simulink model "AUAV3_WITH_SLUGS_SENSOR_AND_CONTROLLER"  (Simulink 8.5)
settings: Solver=FixedStepDiscrete  StartTime=0.0  StopTime=10.0  FixedStep=T  RelTol=1e-3
PreLoadFcn:
  | T = 0.0025;
  | MavlinkBus;
  | 
  | % Baro Altitude Computation
  | % =========================
  | basePressure = 98192.64;
  | baseTemp = 288.215;
  | lapseRate = -0.00198122;
  | baseHeight = 0;
  | 
  | mcuInit
values from neighbouring files (symbols this model uses):
  apSampleTime = 0.01    [mcuInit.m]
  latlong_WP = 1    [mcuInit.m]
  mavlink_gps_raw_int_t = Simulink.Bus    [MavlinkBus.m]    (also in MavlinkBusMarcello.m)
  mavlink_raw_imu_t = Simulink.Bus    [MavlinkBus.m]    (also in MavlinkBusMarcello.m)
  mavlink_scaled_pressure_t = Simulink.Bus    [MavlinkBus.m]    (also in MavlinkBusMarcello.m)
  mavlink_sys_status_t = Simulink.Bus    [MavlinkBus.m]    (also in MavlinkBusMarcello.m)
  Xpoints = [0 0]    [mcuInit.m]
  Ypoints = [0 0]    [mcuInit.m]
  Zpoints = [0 0]    [mcuInit.m]
undefined symbols (not defined in the file or in its folder): A0, A14, A15, A2, A3, A5, A6, accBiasRateLimit, altLatLon, B0, bankCommandLimit, barAdjust, baroCutoff, baroCutTemp, C3, cubeAccelGain16405, cubeGyroGain16405, cubeMagGain16405, D0, D11, D13, D8, daLimit, data, daTrimMax, daTrimMin, deLimit, deTrimMax, deTrimMin, drLimit, drTrimMax, drTrimMin, dtLimit, dtTrimMax, dtTrimMin, F2, F3, G0, G15, gaind, GS_location, gyroBiasRateLimit, IC1max, IPStar, ISA_g, maxAcc, MaxDwnPthStar, maxDynPressure, maxEta, OC1max, P112, P127, P16, P21, P30, P31, P51, P64, P72, P75 ... (+39)
undefined symbols (not defined in the file): baroOffset, baroScale, barTGain1, barTGain2, barTMean1, barTMean2, bda, bde, bdr, bdt, bICda, bICde, bICdr, bICdt, derivativesConstant, lowRateSensorCutoff, mainSensorCutoff, mda, mde, mdr, mdt, mICda, mICde, mICdr, mICdt, pitotOffset, pitotScale, pitTGain1, pitTGain2, pitTMean1, pitTMean2, powerOffset, powerScale, pressureSensorCutoff, tempOffset, tempScale, vzCutoff, xCutoff, yCutoff
libraries: MCHP_Blockset x147, simulink x78, SLUGS_Library x31, aerolibconvert2 x6, aerolibutil x4, aerolibtransform2 x3, dspmtrx3 x2, aerolibobsolete x2
(part 3 of 12)

== system AUAV3_WITH_SLUGS_SENSOR_AND_CONTROLLER/Servo In Out ==
  Bias : Bias  Bias=-round(IC1max/2)
  Bias1 : Bias  Bias=-round(IC1max/2)
  Bias2 : Bias  Bias=+round(IC1max/2)
  Bias3 : Bias  Bias=+round(IC1max/2)
  Data Type Conversion2 : DataTypeConversion  OutDataTypeStr=uint16  ConvertRealWorld=Stored Integer (SI)  RndMeth=Simplest
  Data Type Conversion3 : DataTypeConversion  OutDataTypeStr=uint16  ConvertRealWorld=Stored Integer (SI)  RndMeth=Simplest
  Data Type Conversion4 : DataTypeConversion  OutDataTypeStr=int16  ConvertRealWorld=Stored Integer (SI)  RndMeth=Simplest
  Data Type Conversion5 : DataTypeConversion  OutDataTypeStr=int16  ConvertRealWorld=Stored Integer (SI)  RndMeth=Simplest
  Input Capture RC Receiver1 : MCHP_Blockset/Pulse Input//Output/Input Capture  IntPriority=7  Channel="[1     2     3     4     5     6]"  Channel_OLD="[1  2  3  4  5  6]"  PIN_IC1=Dynamic Options  PIN_IC1_TXT=D0 / P64 / Pin[72]  PIN_IC2=Dynamic Options  PIN_IC2_TXT=D8 / P72 / Pin[68]  PIN_IC3=Dynamic Options  PIN_IC3_TXT=D11 / P75 / Pin[71]  PIN_IC4=Dynamic Options  PIN_IC4_TXT=A15 / P31 / Pin[67]  PIN_IC5=Dynamic Options  PIN_IC5_TXT=A5 / P21 / Pin[61]  PIN_IC6=Dynamic Options  PIN_IC6_TXT=A14 / P30 / Pin[66]  PIN_IC7=Dynamic Options  PIN_IC7_TXT=A0 / P16 / Pin[17]  PIN_IC8=Dynamic Options  PIN_IC8_TXT=A0 / P16 / Pin[17]  PIN_IC9=Dynamic Options  PIN_IC9_TXT=A0 / P16 / Pin[17]  PIN_IC10=Dynamic Options  PIN_IC10_TXT=A0 / P16 / Pin[17]  PIN_IC11=Dynamic Options  PIN_IC11_TXT=A0 / P16 / Pin[17]  PIN_IC12=Dynamic Options  PIN_IC12_TXT=A0 / P16 / Pin[17]  PIN_IC13=Dynamic Options  PIN_IC13_TXT=A0 / P16 / Pin[17]  PIN_IC14=Dynamic Options  PIN_IC14_TXT=A0 / P16 / Pin[17]  PIN_IC15=Dynamic Options  PIN_IC15_TXT=A0 / P16 / Pin[17]  PIN_IC16=Dynamic Options  PIN_IC16_TXT=A0 / P16 / Pin[17]  Channel_UP_Down_Periode="[1     1     1     1     1     1]"  MaxChannel="[0.003   0.003   0.003   0.003   0.003   0.003]"  SafeMarge="[0     0     0     0     0     0]"  MaxChannelValue="2.^[ 14.680  14.680  14.680  14.680  14.680  14.680]  =>  [26249  26249  26249  26249  26249  26249]"  ICxmax="[26249  26249  26249  26249  26249  26249]"  Timer="[1  1  1  1  1  1]"  ChangeDetected="[0     0     0     0     0     0]"  ChangeDetectedPortRef=3  SampleTime=.01  Status=OK  MCHP_PORT={Input Capture 1}{IC1}6:0:P64;{Input Capture 2}{IC2}6:0:P72;{Input Capture 3}{IC3}6:0:P75;{Input Capture 4}{IC4}6:0:P31;{Input Capture 5}{IC5}6:0:P21;{Input Capture 6}{IC6}6:0:P30;  MCHP_TIMER_REQUEST="{Input Capture 1}{IC1}6:0:1:0:[1  2  3  4  5]:210000;{Input Capture 1}{IC1}6:0:1:0:[1  2  3  4  5]:210000;{Input Capture 1}{IC1}6:0:1:0:[1  2  3  4  5]:210000;{Input Capture 1}{IC1}6:0:1:0:[1  2  3  4  5]:210000;{Input Capture 1}{IC1}6:0:1:0:[1  2  3  4  5]:210000;{Input Capture 1}{IC1}6:0:1:0:[1  2  3  4  5]:210000;"  MCHP_TIMER_RESULT=[1 26249.000000000011 ;1 26249.000000000011 ;1 26249.000000000011 ;1 26249.000000000011 ;1 26249.000000000011 ;1 26249.000000000011 ]  MCHP_MASTERLINK=|
      | AUAV3_WITH_SLUGS_SENSOR_AND_CONTROLLER/Microchip Master
      | AUAV V3 Board
      | Busy Flag on D2 (RA6)
  Mixing : Subsystem
  Output Compare - HW Drive Servo motor : MCHP_Blockset/Pulse Input//Output/Output Compare - HW  Channel="[1     2]"  Channel_OLD="[1     2]"  PIN_OC1=Dynamic Options  PIN_OC1_TXT=G0 / P112 / Pin[90]  PIN_OC2=Dynamic Options  PIN_OC2_TXT=E0 / P80 / Pin[93]  PIN_OC3=Dynamic Options  PIN_OC3_TXT=D0 / P64 / Pin[72]  PIN_OC4=Dynamic Options  PIN_OC4_TXT=D0 / P64 / Pin[72]  PIN_OC5=Dynamic Options  PIN_OC5_TXT=D0 / P64 / Pin[72]  PIN_OC6=Dynamic Options  PIN_OC6_TXT=D0 / P64 / Pin[72]  PIN_OC7=Dynamic Options  PIN_OC7_TXT=D0 / P64 / Pin[72]  PIN_OC8=Dynamic Options  PIN_OC8_TXT=D0 / P64 / Pin[72]  PIN_OC9=Dynamic Options  PIN_OC9_TXT=D0 / P64 / Pin[72]  PIN_OC10=Dynamic Options  PIN_OC10_TXT=D0 / P64 / Pin[72]  PIN_OC11=Dynamic Options  PIN_OC11_TXT=D0 / P64 / Pin[72]  PIN_OC12=Dynamic Options  PIN_OC12_TXT=D0 / P64 / Pin[72]  PIN_OC13=Dynamic Options  PIN_OC13_TXT=D0 / P64 / Pin[72]  PIN_OC14=Dynamic Options  PIN_OC14_TXT=D0 / P64 / Pin[72]  PIN_OC15=Dynamic Options  PIN_OC15_TXT=D0 / P64 / Pin[72]  PIN_OC16=Dynamic Options  PIN_OC16_TXT=D0 / P64 / Pin[72]  PIN_OCFA=Dynamic Options  PIN_OCFA_TXT=A0 / P16 / Pin[17]  PIN_OCFB=Dynamic Options  PIN_OCFB_TXT=A0 / P16 / Pin[17]  PIN_OCFC=Dynamic Options  PIN_OCFC_TXT=A0 / P16 / Pin[17]  Channel_UP_Down_Periode="[5     5]"  PulseTrig=Single pulse triggered by block execution  InputPeriod=are set to the Max time (constant below)  MaxChannel="[0.003   0.003]"  MaxChannelUnique=.0001  MaxChannelValue="2.^[ 14.680  14.680]  =>  [26249  26249]"  OCxmax="[26249  26249]"  Timer="[1  1]"  SampleTime=.01  MCHP_PORT={Output Compare 1}{OC1}7:1:P112;{Output Compare 2}{OC2}7:1:P80;  MCHP_TIMER_REQUEST="{Output Compare 1}{OC1}7:0:1:0:[1  2  3  4  5]:210000;{Output Compare 1}{OC1}7:0:1:0:[1  2  3  4  5]:210000;"  MCHP_TIMER_RESULT=[1 26249.000000000011 ;1 26249.000000000011 ]  MCHP_MASTERLINK=|
      | AUAV3_WITH_SLUGS_SENSOR_AND_CONTROLLER/Microchip Master
      | AUAV V3 Board
      | Busy Flag on D2 (RA6)
  Saturation : Saturate  UpperLimit=OC1max*2.2/3  LowerLimit=OC1max*0.8/3  RndMeth=Simplest
  Saturation1 : Saturate  UpperLimit=OC1max*2.2/3  LowerLimit=OC1max*0.8/3  RndMeth=Simplest
  Out1 : Outport
  Out2 : Outport  Port=2
  Out3 : Outport  Port=3
  Out4 : Outport  Port=4
  wires:
  Input Capture RC Receiver1/1 -> Data Type Conversion4/1  "cmd PITCH raw"
  Input Capture RC Receiver1/4 -> Data Type Conversion5/1  "cmd ROLL raw"
  Bias/1 -> Mixing/1(Pitch)
  Bias1/1 -> Mixing/2(Roll)
  Bias2/1 -> Data Type Conversion2/1
  Bias3/1 -> Data Type Conversion3/1
  Saturation1/1 -> Output Compare - HW Drive Servo motor/2
  Saturation/1 -> Output Compare - HW Drive Servo motor/1
  Mixing/2(Cmd Servo Right) -> Bias3/1
  Mixing/1(Cmd Servo Left) -> Bias2/1
  Data Type Conversion4/1 -> Bias/1
  Data Type Conversion5/1 -> Bias1/1
  Data Type Conversion3/1 -> Saturation1/1
  Data Type Conversion2/1 -> Saturation/1
  Input Capture RC Receiver1/2 -> Out1/1
  Input Capture RC Receiver1/3 -> Out2/1
  Input Capture RC Receiver1/5 -> Out3/1
  Input Capture RC Receiver1/6 -> Out4/1

== system AUAV3_WITH_SLUGS_SENSOR_AND_CONTROLLER/Trim Vals [updated 4.28.16] ==
  Bufffer IC : Subsystem
  Control Surfaces [dT dA dR dE] : Selector  InputPortWidth=5  Indices=[1 2 4 3]
  Control Surface Input : Subsystem
  "Convert to Microseconds " : Subsystem
  Detect Transition High to Low : Subsystem
  Failsafe : Selector  InputPortWidth=5  Indices=[5]
  Grab I.C. : Subsystem  TreatAsAtomicUnit=on
  Manual or Auto? [navSupport.c] [updated 4.28.16] : MCHP_Blockset/User Functions/C Function Call  ParseFilesChkbx=off  ListFunctions1=Custom Function  Function1=extern uint8_T isApManual(uint16_T u1);  AddHeaderDeclaration=on  Function1Type=when block is updated (default)  FctReturnBlockOut=on  Fct1BlockOut=y1  DataCollected=0  ORDERING=None  SampleTime=-1  MCHP_MASTERLINK=|  PinDigitalInput=[]  PinDigitalOutput=[]  PinAnalogInput=[]
      | AUAV3_WITH_SLUGS_SENSOR_AND_CONTROLLER/Microchip Master
      | AUAV V3 Board
      | Busy Flag on D2 (RA6)
  Mean Filter the Transition : Subsystem
  dT Trim : Outport
  dA Trim : Outport  Port=2
  dR Trim : Outport  Port=3
  dE Trim : Outport  Port=4
  Pil Console : Outport  Port=5
  Manual? : Outport  Port=6
  V/I Sensor : Outport  Port=7
  wires:
  Manual or Auto? [navSupport.c] [updated 4.28.16]/1 -> Detect Transition High to Low/1(Switch), Manual?/1
  Control Surface Input/1(Pilot Console) -> Control Surfaces [dT dA dR dE]/1, Failsafe/1
  Control Surfaces [dT dA dR dE]/1 -> Pil Console/1, Bufffer IC/1(Pilot Console)
  Bufffer IC/1(dT_buf) -> Grab I.C./1(dT_buf)
  Bufffer IC/2(dA_buf) -> Grab I.C./2(dA_buf)
  Bufffer IC/3(dR_buf) -> Grab I.C./3(dR_buf)
  Bufffer IC/4(dE_buf) -> Grab I.C./4(dE_buf)
  Grab I.C./4(dE_trim (rad)) -> dE Trim/1
  Grab I.C./3(dR_trim (rad)) -> dR Trim/1
  Grab I.C./2(dA_trim (rad)) -> dA Trim/1
  Grab I.C./1(dT_trim (abs)) -> dT Trim/1
  Detect Transition High to Low/1(Transition) -> Grab I.C./Enable
  Failsafe/1 -> "Convert to Microseconds "/1(IC)
  "Convert to Microseconds "/1(uS) -> Mean Filter the Transition/1(Failsafe)
  Control Surface Input/2(Voltage/Current Sensor) -> V/I Sensor/1
  Mean Filter the Transition/1(filtered) -> Manual or Auto? [navSupport.c] [updated 4.28.16]/1

== system AUAV3_WITH_SLUGS_SENSOR_AND_CONTROLLER/Update PWM Commands and Send Telemetry [updated 4.27.16] ==
  PWM(rad) [dT dA dR dE] : Inport
  Pilot Console (IC) [dT dA dR dE] : Inport  Port=2
  Euler_rot : Inport  Port=3
  PQR_rot : Inport  Port=4
  Manual? : Inport  Port=5
  VI : Inport  Port=6
  Convert to Microseconds : Subsystem
  Create Telemetry Sentence [mavlinkCommsControlMcu.c] : MCHP_Blockset/User Functions/C Function Call  ParseFilesChkbx=off  ListFunctions1=Custom Function  Function1=extern void prepareTelemetryMavlink(uint8_T* y1);  AddHeaderDeclaration=on  Function1Type=when block is updated (default)  FctReturnBlockOut=on  Fct1BlockOut=y1  DataCollected=0  ORDERING=Input  SampleTime=0.04  MCHP_MASTERLINK=|  PinDigitalInput=[]  PinDigitalOutput=[]  PinAnalogInput=[]
      | AUAV3_WITH_SLUGS_SENSOR_AND_CONTROLLER/Microchip Master
      | AUAV V3 Board
      | Busy Flag on D2 (RA6)
  Demux : Demux
  Generate PWM Signals Based on the Control Type : Subsystem
  Navigation Mode [navSupport.c] : MCHP_Blockset/User Functions/C Function Call  ParseFilesChkbx=off  ListFunctions1=Custom Function  Function1=extern uint8_T getNavMode();  AddHeaderDeclaration=on  Function1Type=when block is updated (default)  FctReturnBlockOut=on  DataCollected=0  ORDERING=None  SampleTime=0.01  MCHP_MASTERLINK=|  PinDigitalInput=[]  PinDigitalOutput=[]  PinAnalogInput=[]
      | AUAV3_WITH_SLUGS_SENSOR_AND_CONTROLLER/Microchip Master
      | AUAV V3 Board
      | Busy Flag on D2 (RA6)
  PWM High Speed : MCHP_Blockset/PWM IO/PWM High Speed  pop1=[1]  chk1="[1  1  1  0]"  chkHL1="[1  1  1  1  0  0  1 ; 1  1  1  1  0  0  1]"  maxP1="[0.001       0.001       0.001       0.001       0.001       0.001       0.001 ; 0.001       0.001      1e-006       0.001       0.001       0.001       0.001]"  InitP2="[0.001       0.001       0.001       0.001       0.001       0.001       0.001 ; 0.001       0.001       0.001       0.001       0.001       0.001       0.001]"  chkP2="[0  0  0  0  1  1  1 ; 1  0  0  1  1  1  1]"  InitDC="[0.0005       0.0004       0.0003        0.001        0.001        0.001           50 ; 0.001        0.001        0.001        0.001        0.001        0.001           50]"  chkDC="[1  1  1  1  1  1  1 ; 0  0  0  1  1  1  1]"  InitPh="[0           0           0       0.001       0.001       0.001       0.001 ; 0           0           0       0.001       0.001       0.001       0.001]"  chkPh="[0  0  0  1  1  1  1 ; 0  0  0  1  1  1  1]"  edSEvTrigx={'0.0006','-1','-1','-1','-1','-1','-1'}  chkSEvTrigx="[0  0  0  0  1  1  1]"  popFlt="[1  1  1  1  1  1  1]"  popFltPin="[48  48  48  48  48  48  48]"  popFltPinRp="[1  1  1  1  1  1  1]"  popFltActivH="[1  2  1  1  1  1  1]"  popFltForceH="[2  2  2  2  2  2  2]"  popFltForceL="[1  1  1  1  1  1  1]"  chkFltBlkOut="[0  0  0  0  0  0  0]"  popDT="[3  3  3  3  3  3  3]"  edDTRx="[0.02      1e-005       0.001      1e-005      1e-005      1e-005      1e-005]"  edAltDTRx="[1e-005      0.0001      1e-005      1e-005      1e-005      1e-005      1e-005]"  S_INPUT="[5  5  5  5]"  S_OUTPUT=[]  ADC_VARTRIG={PWM Generator 1 Primary Trigger;1}{PWM Generator 2 Primary Trigger;3}{PWM Generator 3 Primary Trigger;5}{PWM Generator 4 Primary Trigger;7}  SampleTime=-1  ORDERING=None  MCHP_PORT={PWM1H}{PWM1H}4:4:E0;{PWM1L}{PWM1L}4:4:E1;{PWM2H}{PWM2H}4:4:E2;{PWM2L}{PWM2L}4:4:E3;{PWM3H}{PWM3H}4:4:E4;{PWM3L}{PWM3L}4:4:E5;{PWM4H}{PWM4H}4:4:E6;{PWM4L}{PWM4L}4:4:E7;  MCHP_MASTERLINK=|
      | AUAV3_WITH_SLUGS_SENSOR_AND_CONTROLLER/Microchip Master
      | AUAV V3 Board
      | Busy Flag on D2 (RA6)
  Rate Transition : RateTransition
  Send Data to Radio Modem [mavlinkCommsControlMcu.c] : MCHP_Blockset/User Functions/C Function Call  ParseFilesChkbx=off  ListFunctions1=Custom Function  Function1=extern void send2GS(uint8_T* u1);  AddHeaderDeclaration=on  Function1Type=when block is updated (default)  FctReturnBlockOut=on  Fct1BlockOut=y1  DataCollected=0  ORDERING=None  SampleTime=0.04  MCHP_MASTERLINK=|  PinDigitalInput=[]  PinDigitalOutput=[]  PinAnalogInput=[]
      | AUAV3_WITH_SLUGS_SENSOR_AND_CONTROLLER/Microchip Master
      | AUAV V3 Board
      | Busy Flag on D2 (RA6)
  Update Euler Angles [updateControlMcu.c] : MCHP_Blockset/User Functions/C Function Call  ParseFilesChkbx=off  ListFunctions1=Custom Function  Function1=extern void updateEuler(real32_T* u1);  AddHeaderDeclaration=on  Function1Type=when block is updated (default)  Fct1BlockIn=u1  FctReturnBlockOut=on  DataCollected=0  ORDERING=Input & Output  SampleTime=0.01  MCHP_MASTERLINK=|  PinDigitalInput=[]  PinDigitalOutput=[]  PinAnalogInput=[]
      | AUAV3_WITH_SLUGS_SENSOR_AND_CONTROLLER/Microchip Master
      | AUAV V3 Board
      | Busy Flag on D2 (RA6)
  Update PQR [updateControlMcu.c] : MCHP_Blockset/User Functions/C Function Call  ParseFilesChkbx=off  ListFunctions1=Custom Function  Function1=extern void updatePQR(real32_T* u1);  AddHeaderDeclaration=on  Function1Type=when block is updated (default)  Fct1BlockIn=u1  FctReturnBlockOut=on  DataCollected=0  ORDERING=Input & Output  SampleTime=0.01  MCHP_MASTERLINK=|  PinDigitalInput=[]  PinDigitalOutput=[]  PinAnalogInput=[]
      | AUAV3_WITH_SLUGS_SENSOR_AND_CONTROLLER/Microchip Master
      | AUAV V3 Board
      | Busy Flag on D2 (RA6)
  Update Voltage/Current Sensor [updateControlMcu.c] : MCHP_Blockset/User Functions/C Function Call  ParseFilesChkbx=off  ListFunctions1=Custom Function  Function1=extern void updateVISensor(uint16_T* u1);  AddHeaderDeclaration=on  Function1Type=when block is updated (default)  Fct1BlockIn=u1  FctReturnBlockOut=on  DataCollected=0  ORDERING=Input & Output  SampleTime=0.01  MCHP_MASTERLINK=|  PinDigitalInput=[]  PinDigitalOutput=[]  PinAnalogInput=[]
      | AUAV3_WITH_SLUGS_SENSOR_AND_CONTROLLER/Microchip Master
      | AUAV V3 Board
      | Busy Flag on D2 (RA6)
  Update the Euler Angles [updateControlMcu.c] : MCHP_Blockset/User Functions/C Function Call  ParseFilesChkbx=off  ListFunctions1=Custom Function  Function1=extern void updatePWM(uint16_T* u1);  AddHeaderDeclaration=on  Function1Type=when block is updated (default)  Fct1BlockIn=u1  FctReturnBlockOut=on  DataCollected=0  ORDERING=Output  SampleTime=0.01  MCHP_MASTERLINK=|  PinDigitalInput=[]  PinDigitalOutput=[]  PinAnalogInput=[]
      | AUAV3_WITH_SLUGS_SENSOR_AND_CONTROLLER/Microchip Master
      | AUAV V3 Board
      | Busy Flag on D2 (RA6)
  "[dR dE dA dT]" : Selector  InputPortWidth=4  Indices=[3 4 2 1]
  wires:
  "[dR dE dA dT]"/1 -> Demux/1
  Demux/1 -> PWM High Speed/1
  Demux/2 -> PWM High Speed/2
  Demux/3 -> PWM High Speed/3
  Demux/4 -> PWM High Speed/4
  Generate PWM Signals Based on the Control Type/1(PWM) -> "[dR dE dA dT]"/1, Convert to Microseconds/1(PWM)  "[dT dA dR dE]"
  PWM(rad) [dT dA dR dE]/1 -> Generate PWM Signals Based on the Control Type/1(PWM(rad))
  Pilot Console (IC) [dT dA dR dE]/1 -> Generate PWM Signals Based on the Control Type/2(Pilot Console (IC))
  Convert to Microseconds/1(uS) -> Update the Euler Angles [updateControlMcu.c]/1
  Manual?/1 -> Generate PWM Signals Based on the Control Type/3(isManual?)
  Navigation Mode [navSupport.c]/1 -> Generate PWM Signals Based on the Control Type/4(Nav Mode)
  Euler_rot/1 -> Update Euler Angles [updateControlMcu.c]/1
  Update the Euler Angles [updateControlMcu.c]/1 -> Update Euler Angles [updateControlMcu.c]/2
  PQR_rot/1 -> Update PQR [updateControlMcu.c]/1
  Update Euler Angles [updateControlMcu.c]/1 -> Update PQR [updateControlMcu.c]/2
  VI/1 -> Update Voltage/Current Sensor [updateControlMcu.c]/1
  Update PQR [updateControlMcu.c]/1 -> Update Voltage/Current Sensor [updateControlMcu.c]/2
  Create Telemetry Sentence [mavlinkCommsControlMcu.c]/1 -> Send Data to Radio Modem [mavlinkCommsControlMcu.c]/1
  Update Voltage/Current Sensor [updateControlMcu.c]/1 -> Rate Transition/1
  Rate Transition/1 -> Create Telemetry Sentence [mavlinkCommsControlMcu.c]/1

== system AUAV3_WITH_SLUGS_SENSOR_AND_CONTROLLER/get Nav Vars [updated 4.28.16] ==
  Attitude : Inport
  Accel : Inport  Port=2
  Accel. Bias : Inport  Port=3
  Angle Conversion : aerolibconvert2/Angle Conversion  IU=deg  OU=rad
  Constant1 : Constant  Value=PAR_CONFIG_ROLL_R  OutDataTypeStr=uint8
  Constant7 : Constant  Value=PAR_CONFIG_YAW_R  OutDataTypeStr=uint8
  Demux : Demux  Outputs=3
  Direction Cosine Matrix to Rotation Angles : aerolibtransform2/Direction Cosine Matrix to Rotation Angles  rotationOrder=ZYX  lim=Default
      settings: AttributesFormatString=Rotation Order: %<rotationOrder>
  Embedded MATLAB Function1 : MATLAB Function  TreatAsAtomicUnit=on
  Euler : Selector  InputPortWidth=6  Indices=[1 2 3]
  Euler Angles to  Direction Cosine Matrix1 : aerolibobsolete/Euler Angles to  Direction Cosine Matrix
  Euler Angles to  Direction Cosine Matrix2 : aerolibobsolete/Euler Angles to  Direction Cosine Matrix
  Get Range of Values [navSupport.c] [updated 4.27.16] : MCHP_Blockset/User Functions/C Function Call  ParseFilesChkbx=off  ListFunctions1=Custom Function  Function1=extern void getRangeOfParams(uint8_T u1, uint8_T u2, real32_T* y1);  AddHeaderDeclaration=on  Function1Type=when block is updated (default)  Fct1BlockIn=u1 u2  FctReturnBlockOut=on  Fct1BlockOut=y1  DataCollected=0  ORDERING=None  SampleTime=0.01  MCHP_MASTERLINK=|  PinDigitalInput=[]  PinDigitalOutput=[]  PinAnalogInput=[]
      | AUAV3_WITH_SLUGS_SENSOR_AND_CONTROLLER/Microchip Master
      | AUAV V3 Board
      | Busy Flag on D2 (RA6)
  Math Function : Math  Operator=transpose  SaturateOnIntegerOverflow=on
  Product{,1..3} (4 alike) : Product  Multiplication=Matrix(*)  RndMeth=Zero
  Rates : Selector  InputPortWidth=6  Indices=[4 5 6]
  Selector : Selector  InputPortWidth=6  Indices=[1 2 5 6]
  Selector1 : Selector  InputPortWidth=3  Indices=[2]
  Sum : Sum  Inputs=+|+
  myMux Fun1 : MATLAB Function  TreatAsAtomicUnit=on
  myMux Fun2 : MATLAB Function  TreatAsAtomicUnit=on
  "[phi the q r]" : Outport
  Euler Rot : Outport  Port=2
  PQR Rot : Outport  Port=3
  Yb Accel : Outport  Port=4
  wires:
  Selector/1 -> "[phi the q r]"/1
  Euler/1 -> Euler Angles to  Direction Cosine Matrix2/1
  Euler Angles to  Direction Cosine Matrix2/1 -> Product/2
  Euler Angles to  Direction Cosine Matrix1/1 -> Math Function/1
  Angle Conversion/1 -> Euler Angles to  Direction Cosine Matrix1/1
  Product/1 -> Direction Cosine Matrix to Rotation Angles/1
  Rates/1 -> Product1/2
  myMux Fun1/1(y) -> Euler Rot/1, myMux Fun2/1(u1)
  Product1/1 -> myMux Fun2/2(u2), PQR Rot/1
  myMux Fun2/1(y) -> Selector/1
  Math Function/1 -> Product/1, Product1/1, Product2/1, Product3/1
  Accel/1 -> Product2/2
  Accel. Bias/1 -> Product3/2
  Product2/1 -> Sum/1
  Product3/1 -> Sum/2
  Sum/1 -> Selector1/1
  Selector1/1 -> Yb Accel/1
  Demux/1 -> Embedded MATLAB Function1/1(u)
  Direction Cosine Matrix to Rotation Angles/1 -> Demux/1
  Demux/2 -> myMux Fun1/2(u2)
  Demux/3 -> myMux Fun1/1(u1)
  Embedded MATLAB Function1/1(y) -> myMux Fun1/3(u3)
  Attitude/1 -> Euler/1, Rates/1
  Constant1/1 -> Get Range of Values [navSupport.c] [updated 4.27.16]/1
  Constant7/1 -> Get Range of Values [navSupport.c] [updated 4.27.16]/2
  Get Range of Values [navSupport.c] [updated 4.27.16]/1 -> Angle Conversion/1

== system AUAV3_WITH_SLUGS_SENSOR_AND_CONTROLLER/Control Surface Input/Convert to Microseconds  ==
  IC : Inport
  Convert to  Microseconds : Gain  Gain=0.2
  Data Type Conversion : DataTypeConversion  OutDataTypeStr=uint16
  uS : Outport
  wires:
  Convert to  Microseconds/1 -> Data Type Conversion/1
  IC/1 -> Convert to  Microseconds/1
  Data Type Conversion/1 -> uS/1

== system AUAV3_WITH_SLUGS_SENSOR_AND_CONTROLLER/Inner Loop/ Navigation/Compute psi_dot_m ==
  r_m : Inport
  phi_m : Inport  Port=2
  q_m : Inport  Port=3
  Product : Product  SampleTime=apSampleTime  RndMeth=Zero
  Product1 : Product  SampleTime=apSampleTime  RndMeth=Zero
  Protect NaNs : Subsystem
  Subtract : Sum  Inputs=2
  dsPIC_cos : Subsystem  AncestorBlock=SLUGS_Library/dsPIC_cos
  dsPIC_sin : Subsystem  AncestorBlock=SLUGS_Library/dsPIC_sin
  psi_dot_m : Outport
  wires:
  q_m/1 -> Product1/1
  Subtract/1 -> Protect NaNs/1(In1)
  phi_m/1 -> dsPIC_sin/1(x), dsPIC_cos/1(u)
  r_m/1 -> Product/1
  Product1/1 -> Subtract/2
  Product/1 -> Subtract/1
  dsPIC_sin/1(sin(x)) -> Product1/2
  dsPIC_cos/1(cos(u)) -> Product/2
  Protect NaNs/1(Out1) -> psi_dot_m/1

== system AUAV3_WITH_SLUGS_SENSOR_AND_CONTROLLER/Inner Loop/ Navigation/L1 Output Feedback Controller With  Projection Operator ==
  psi_dot_m : Inport
  m : Inport  Port=2
  omega : Inport  Port=3
  gamma : Inport  Port=4
  psi_dot_c : Inport  Port=5
  Enable : EnablePort  StatesWhenEnabling=reset  ShowOutputPort=on
  Constant : Constant  Value=2  OutDataTypeStr=single
  Constant1 : Constant  OutDataTypeStr=single
  Control  Law : Subsystem
      mask Display:
      | droots([],'-a','a')
      | port_label('input',1,'a')
      | port_label('input',2,'u')
      | port_label('output',1,'y')
  Gain : Gain  Gain=-1  OutDataTypeStr=Inherit: Same as input
  Integer Delay : Delay  DelayLength=1  InputProcessing=Inherited  SampleTime=.01
  Integer Delay1 : Delay  DelayLength=1  InputProcessing=Inherited  SampleTime=.01
  Logical Operator : Logic  Operator=NOT  AllPortsSameDT=off  OutDataTypeStr=uint(8)
  Projection : Product  OutDataTypeStr=single  SampleTime=apSampleTime  RndMeth=Zero
  Projection Operator : Subsystem
  Protect NaNs : Subsystem
  Protect NaNs2 : Subsystem
  Psi Dot  Limit : Saturate  UpperLimit=1  LowerLimit=-1  SampleTime=apSampleTime
  State Predictor : Subsystem
      mask Display:
      | droots([],'-a','a')
      | port_label('input',1,'a')
      | port_label('input',2,'u')
      | port_label('output',1,'y')
  Sum2 : Sum  Inputs=|++  OutDataTypeStr=single  SampleTime=apSampleTime
  Sum3 : Sum  Inputs=-+|  OutDataTypeStr=single  SampleTime=apSampleTime
  Sum4 : Sum  Inputs=+-|  OutDataTypeStr=single  SampleTime=apSampleTime
  Trapezoidal Integrator : Subsystem  AncestorBlock=SLUGS_Library/Control Blocks/PID Controller w//Anti-Windup/Trapezoidal Integrator  mask{T=apSampleTime, upperLimit=2, lowerLimit=-2}
      mask prompts: T "Sample Time"; upperLimit "Upper Saturation"; lowerLimit "Lower Saturation"
  psi_dot_ad : Outport
  wires:
  Integer Delay/1 -> Sum4/1  "psi_dot_c"
  State Predictor/1(y) -> Sum3/2
  Gain/1 -> Projection Operator/4(y)
  m/1 -> State Predictor/1(a)
  Sum2/1 -> Protect NaNs2/1(In1)
  psi_dot_m/1 -> Protect NaNs/1(In1)  "psi_dot_m"
  Sum3/1 -> Gain/1  "psi_dot_tilde"
  gamma/1 -> Projection/1  "adaptation gain"
  Projection/1 -> Trapezoidal Integrator/1(x)
  psi_dot_c/1 -> Integer Delay/1  "psi_dot_c"
  omega/1 -> Control  Law/1(a)
  Control  Law/1(y) -> Sum4/2  "sigma_hat_fil"
  Sum4/1 -> Psi Dot  Limit/1  "psi_ad"
  Projection Operator/1("Proj(the, y)") -> Projection/2  "Proj"
  Constant/1 -> Projection Operator/1(Theta Max)
  Constant1/1 -> Projection Operator/2(Eps 0)
  Integer Delay1/1 -> Sum2/2, Projection Operator/3(Theta)
  Enable/1 -> Logical Operator/1
  Logical Operator/1 -> Trapezoidal Integrator/2(Reset)
  Trapezoidal Integrator/1(Int(x)) -> Control  Law/2(u), Integer Delay1/1  "sigma_hat"
  Protect NaNs2/1(Out1) -> State Predictor/2(u)
  Protect NaNs/1(Out1) -> Sum3/1
  Psi Dot  Limit/1 -> psi_dot_ad/1, Sum2/1

== system AUAV3_WITH_SLUGS_SENSOR_AND_CONTROLLER/Inner Loop/ Navigation/Lateral Channel Encaps [updated 4.28.16] ==
  r_m : Inport
  Manual? : Inport  Port=2
  Yaw Damp  PID Gains : Inport  Port=3
  dR Trim : Inport  Port=4
  psi_dot_c_noNav : Inport  Port=5
  U_m : Inport  Port=6
  phi_m : Inport  Port=7
  Roll PID Gains : Inport  Port=8
  dA Trim : Inport  Port=9
  nav_phi_c : Inport  Port=10
  psi_dot_ad : Inport  Port=11  SampleTime=apSampleTime
  L1OnOff : Inport  Port=12
  Enable SS Comp : Inport  Port=13
  Ayb : Inport  Port=14
  dR Mix? : Inport  Port=15
  dR Mix gain : Inport  Port=16
  isPassthrough : Inport  Port=17
  Lateral Channel : Subsystem  AncestorBlock=SLUGS_Library/Control Blocks/Lateral Channel
  U_m1 : InportShadow  Port=6
  Update Lat. Chan. Commands [navSupport.c] [updated 4.28.16] : MCHP_Blockset/User Functions/C Function Call  ParseFilesChkbx=off  ListFunctions1=Custom Function  Function1=extern void setNavLat(real32_T* u1);  AddHeaderDeclaration=on  Function1Type=when block is updated (default)  Fct1BlockIn=u1  FctReturnBlockOut=on  Fct1BlockOut=y1  DataCollected=0  ORDERING=None  SampleTime=0.01  MCHP_MASTERLINK=|  PinDigitalInput=[]  PinDigitalOutput=[]  PinAnalogInput=[]
      | AUAV3_WITH_SLUGS_SENSOR_AND_CONTROLLER/Microchip Master
      | AUAV V3 Board
      | Busy Flag on D2 (RA6)
  myMux Fun1 : MATLAB Function  TreatAsAtomicUnit=on
  psi_dot_c Select logic1 : Subsystem  AncestorBlock=SLUGS_Library/Control Blocks/psi_dot_c Select logic
  dA : Outport
  dR : Outport  Port=2
  phi_c : Outport  Port=3
  psi_dot_c_4_L1 : Outport  Port=4
  wires:
  Lateral Channel/4(psiDot) -> myMux Fun1/1(u1)
  Lateral Channel/5(rHp) -> myMux Fun1/3(u3)
  dR Trim/1 -> Lateral Channel/4(dR Trim)
  phi_m/1 -> Lateral Channel/7(phi_m)
  r_m/1 -> Lateral Channel/1(r_m)
  Lateral Channel/1(dA) -> dA/1
  Roll PID Gains/1 -> Lateral Channel/8(Roll PID Gains)
  dA Trim/1 -> Lateral Channel/9(dA Trim)
  Enable SS Comp/1 -> Lateral Channel/10(Enable SS Comp)
  Manual?/1 -> Lateral Channel/2(Manual?)
  Ayb/1 -> Lateral Channel/11(Ayb)
  dR Mix gain/1 -> Lateral Channel/13(dR Mix gain)
  Lateral Channel/2(dR) -> dR/1
  Yaw Damp  PID Gains/1 -> Lateral Channel/3(Yaw Damp  PID Gains)
  dR Mix?/1 -> Lateral Channel/12(dR Mix?)
  Lateral Channel/3(phi_c) -> phi_c/1, myMux Fun1/2(u2)
  U_m/1 -> Lateral Channel/6(U_m)
  nav_phi_c/1 -> psi_dot_c Select logic1/5(nav_phi_c)
  U_m1/1 -> psi_dot_c Select logic1/6(U_m)
  psi_dot_ad/1 -> psi_dot_c Select logic1/1(psi_dot_ad)
  L1OnOff/1 -> psi_dot_c Select logic1/2(L1OnOff)
  psi_dot_c_noNav/1 -> psi_dot_c Select logic1/3(psi_dot_c_noNav)
  [psi_dot_c] -> Lateral Channel/5(psi_dot_c)
  psi_dot_c Select logic1/1(psi_dot_c) -> [psi_dot_c]
  psi_dot_c Select logic1/2(psi_dot_c_4_L1) -> psi_dot_c_4_L1/1
  isPassthrough/1 -> psi_dot_c Select logic1/4(IsPassThrough)
  myMux Fun1/1(y) -> Update Lat. Chan. Commands [navSupport.c] [updated 4.28.16]/1

== system AUAV3_WITH_SLUGS_SENSOR_AND_CONTROLLER/Inner Loop/ Navigation/Longitudinal Channel Encaps [updated 4.28.16] ==
  U_c : Inport
  dyn P : Inport  Port=2
  U_hold PID  Gains : Inport  Port=3
  dT_trim : Inport  Port=4
  h_c : Inport  Port=5
  h_m : Inport  Port=6
  he2th PI Gains : Inport  Port=7
  Roll to Height FF : Inport  Port=8
  theta_m : Inport  Port=9
  th2dE PID Gains : Inport  Port=10
  dE_trim : Inport  Port=11
  Manual? : Inport  Port=12
  phi_m : Inport  Port=13
  dt FF Gain : Inport  Port=14
  Constant3 : Constant  Value=[100 100 100]  OutDataTypeStr=single
  Longitudinal Channel : Subsystem  AncestorBlock=SLUGS_Library/Control Blocks/Longitudinal Channel
  Update Long. Chan. Commands [navSupport.c] [updated 4.28.16] : MCHP_Blockset/User Functions/C Function Call  ParseFilesChkbx=off  ListFunctions1=Custom Function  Function1=extern void setNavLong(real32_T* u1);  AddHeaderDeclaration=on  Function1Type=when block is updated (default)  Fct1BlockIn=u1  FctReturnBlockOut=on  Fct1BlockOut=y1  DataCollected=0  ORDERING=None  SampleTime=0.01  MCHP_MASTERLINK=|  PinDigitalInput=[]  PinDigitalOutput=[]  PinAnalogInput=[]
      | AUAV3_WITH_SLUGS_SENSOR_AND_CONTROLLER/Microchip Master
      | AUAV V3 Board
      | Busy Flag on D2 (RA6)
  myMux Fun1 : MATLAB Function  TreatAsAtomicUnit=on
  dE : Outport
  dT : Outport  Port=2
  theta_C : Outport  Port=3
  h_c_in : Outport  Port=4
  U_m : Outport  Port=5
  wires:
  U_c/1 -> Longitudinal Channel/1(U_c)
  dyn P/1 -> Longitudinal Channel/2(dyn P)
  U_hold PID  Gains/1 -> Longitudinal Channel/3(U_hold PID  Gains)
  dT_trim/1 -> Longitudinal Channel/4(dT_trim)
  h_m/1 -> Longitudinal Channel/6(h_m)
  theta_m/1 -> Longitudinal Channel/9(theta_m)
  dE_trim/1 -> Longitudinal Channel/11(dE_trim)
  Manual?/1 -> Longitudinal Channel/12(Manual?)
  he2th PI Gains/1 -> Longitudinal Channel/7(he2th PI Gains)
  Roll to Height FF/1 -> Longitudinal Channel/8(Roll to Height FF)
  th2dE PID Gains/1 -> Longitudinal Channel/10(th2dE PID Gains)
  dt FF Gain/1 -> Longitudinal Channel/14(dt FF Gain)
  h_c/1 -> Longitudinal Channel/5(h_c)
  phi_m/1 -> Longitudinal Channel/13(phi_m)
  Longitudinal Channel/1(dE) -> dE/1  "U"
  Longitudinal Channel/2(dT) -> dT/1
  Longitudinal Channel/3(h_c_in) -> h_c_in/1, myMux Fun1/3(u3)
  Longitudinal Channel/4(U_m) -> U_m/1, myMux Fun1/1(u1)
  Longitudinal Channel/5(theta_C) -> theta_C/1, myMux Fun1/2(u2)
  Constant3/1 -> Longitudinal Channel/15(GS Location)
  myMux Fun1/1(y) -> Update Long. Chan. Commands [navSupport.c] [updated 4.28.16]/1

== system AUAV3_WITH_SLUGS_SENSOR_AND_CONTROLLER/Inner Loop/ Navigation/Navigation Encaps [updated 4.28.16] ==
  Puav : Inport  SampleTime=apSampleTime
  Max WP Idx : Inport  Port=2
  Vxyz : Inport  Port=3  SampleTime=apSampleTime
  T*(m) : Inport  Port=4
  U_c : Inport  Port=5
  WPFly : Inport  Port=6
  TurnLeadTime : Inport  Port=7
  RTB : Inport  Port=8
  Mobile Location : Inport  Port=9
  Follow Mobile? : Inport  Port=10
  MidLvl h_c : Inport  Port=11
  isApManual? : Inport  Port=12
  ISR Scale : Inport  Port=13
  Nav. Mode [navSupport.c] [updated 4.28.16] : MCHP_Blockset/User Functions/C Function Call  ParseFilesChkbx=off  ListFunctions1=Custom Function  Function1=extern uint8_T getNavMode();  AddHeaderDeclaration=on  Function1Type=when block is updated (default)  FctReturnBlockOut=on  Fct1BlockOut=y1[3]  DataCollected=0  ORDERING=None  SampleTime=0.01  MCHP_MASTERLINK=|  PinDigitalInput=[]  PinDigitalOutput=[]  PinAnalogInput=[]
      | AUAV3_WITH_SLUGS_SENSOR_AND_CONTROLLER/Microchip Master
      | AUAV V3 Board
      | Busy Flag on D2 (RA6)
  Nav. Mode [navSupport.c] [updated 4.28.16]1 : MCHP_Blockset/User Functions/C Function Call  ParseFilesChkbx=off  ListFunctions1=Custom Function  Function1=extern void getISRLocation(real32_T* y1);  AddHeaderDeclaration=on  Function1Type=when block is updated (default)  FctReturnBlockOut=on  Fct1BlockOut=y1[3]  DataCollected=0  ORDERING=None  SampleTime=0.01  MCHP_MASTERLINK=|  PinDigitalInput=[]  PinDigitalOutput=[]  PinAnalogInput=[]
      | AUAV3_WITH_SLUGS_SENSOR_AND_CONTROLLER/Microchip Master
      | AUAV V3 Board
      | Busy Flag on D2 (RA6)
  Navigation : Subsystem  AncestorBlock=SLUGS_Library/Navigation/Navigation
  h_c : Outport
  phi_c : Outport  Port=2
  ISR Loc : Outport  Port=3
  "Puav " : Outport  Port=4
  wires:
  T*(m)/1 -> Navigation/2(T*(m))
  WPFly/1 -> Navigation/3(WPFly)
  RTB/1 -> Navigation/4(RTB)
  isApManual?/1 -> Navigation/5(isApManual?)
  Navigation/1(h_c) -> h_c/1
  Navigation/2(phi_c) -> phi_c/1
  Puav/1 -> Navigation/6(Puav)
  Navigation/4("Puav ") -> "Puav "/1
  Max WP Idx/1 -> Navigation/8(Max WP Idx)
  Vxyz/1 -> Navigation/9(Vxyz)
  U_c/1 -> Navigation/10(U_c)
  TurnLeadTime/1 -> Navigation/11(TurnLeadTime)
  Mobile Location/1 -> Navigation/12(Mobile Location)
  Follow Mobile?/1 -> Navigation/13(Follow Mobile?)
  MidLvl h_c/1 -> Navigation/14(MidLvl h_c)
  ISR Scale/1 -> Navigation/15(ISR Scale)
  Navigation/3(ISR Loc) -> ISR Loc/1
  Nav. Mode [navSupport.c] [updated 4.28.16]/1 -> Navigation/1(NavMode)
  Nav. Mode [navSupport.c] [updated 4.28.16]1/1 -> Navigation/7(ISR Location)

== system AUAV3_WITH_SLUGS_SENSOR_AND_CONTROLLER/Inner Loop/ Navigation/Protect NaNs ==
  In1 : Inport
  Integer Delay3 : Delay  DelayLength=1  InputProcessing=Inherited  SampleTime=T
  Relational Operator2 : RelationalOperator  Operator===  OutDataTypeStr=uint(8)
  Switch3 : Switch  Criteria=u2 > Threshold  Threshold=0.3  SampleTime=.01
  Out1 : Outport
  wires:
  Integer Delay3/1 -> Switch3/3
  Switch3/1 -> Out1/1, Integer Delay3/1
  In1/1 -> Relational Operator2/2, Relational Operator2/1, Switch3/1
  Relational Operator2/1 -> Switch3/2

== system AUAV3_WITH_SLUGS_SENSOR_AND_CONTROLLER/Position and Attitude Filter [updated 5.13.16]/Attitude Complimentary Filter COG ==
  A_sens : Inport  PortDimensions=3
  XY Orient : Inport  Port=2  OutDataTypeStr=single
  Gyros : Inport  Port=3  PortDimensions=3
  Vxyd_hat : Inport  Port=4  PortDimensions=3
  acc_bias : Inport  Port=5  PortDimensions=3
  3D Filter : Subsystem  AncestorBlock=SLUGS_Library/Singnal Routing & Conditioning/3D Filter  RTWFcnName=TustinFilter3D  mask{zval=[], pval=[0], kval=1, TSample=0.01}
      mask prompts: zval "Zeros"; pval "Poles"; kval "Gains"; TSample "Sample Time"
      settings: RTWFcnNameOpts=User specified  RTWFileNameOpts=Use function name
      mask Display:
      | droots(zval,pval,kval)
      | port_label('input',1,'3D')
  3x3 Cross Product : aerolibutil/3x3 Cross Product
  3x3 Cross Product1 : aerolibutil/3x3 Cross Product
  3x3 Cross Product2 : aerolibutil/3x3 Cross Product
  Add : Sum  Inputs=++--
  Bias Rate Limiter : RateLimiter  RisingSlewLimit=gyroBiasRateLimit  FallingSlewLimit=-gyroBiasRateLimit  SampleTimeMode=inherited
  Constant1 : Constant  Value=0  OutDataTypeStr=single
  Data Type Conversion : DataTypeConversion  OutDataTypeStr=single
  Demux : Demux  Outputs=3
  Demux1 : Demux  Outputs=3
  "Deriv " : Subsystem
  Direction Cosine Matrix to Rotation Angles : aerolibtransform2/Direction Cosine Matrix to Rotation Angles  rotationOrder=ZYX  lim=Default
      settings: AttributesFormatString=Rotation Order: %<rotationOrder>
  Discrete-Time Integrator1 : DiscreteIntegrator  InitialCondition=q_quat  SampleTime=apSampleTime  LimitOutput=on  UpperSaturationLimit=[1 1 1 1]  LowerSaturationLimit=[-1 -1 -1 -1]
  Embedded MATLAB Function : MATLAB Function  TreatAsAtomicUnit=on
  Gain : Gain  Gain=0.1
  Gain1 : Gain  Gain=30
  Integer Delay : Delay  DelayLength=1  InputProcessing=Inherited
  Mux : Mux  Inputs=3
  Normalize Vector1 : Subsystem  AncestorBlock=SLUGS_Library/Navigation/Normalize Vector
  Normalize Vector2 : Subsystem  AncestorBlock=SLUGS_Library/Navigation/Normalize Vector
  Product1 : Product  Multiplication=Matrix(*)  RndMeth=Zero
  Product2 : Product  Multiplication=Matrix(*)  RndMeth=Zero
  Quaternion Normalize : aerolibutil/Quaternion Normalize
  Quaternions to  Direction Cosine Matrix : aerolibtransform2/Quaternions to  Direction Cosine Matrix
  Submatrix : dspmtrx3/Submatrix  RowSpan=Range of rows  RowStartMode=First  RowStartIndex=1  RowEndMode=Last  RowEndIndex=1  ColSpan=One column  ColStartMode=Last  ColStartIndex=1  ColEndMode=Last  ColEndIndex=1
  Submatrix1 : dspmtrx3/Submatrix  RowSpan=One row  RowStartMode=First  RowStartIndex=1  RowEndMode=Last  RowEndIndex=1  ColSpan=All columns  ColStartMode=Last  ColStartIndex=1  ColEndMode=Last  ColEndIndex=1
  Sum1 : Sum  Inputs=++|
  Sum3 : Sum  Inputs=++|
  Sum4 : Sum  Inputs=++|
  Terminator10 : Terminator
  myMux Fun2 : MATLAB Function  TreatAsAtomicUnit=on
  q dot calc : MATLAB Function  TreatAsAtomicUnit=on
  euler_hat : Outport
  pqr_hat : Outport  Port=2
  Gyro Bias : Outport  Port=3
  RL2B : Outport  Port=4
  wires:
  Bias Rate Limiter/1 -> Gyro Bias/1, Sum3/2
  Product2/1 -> Gain1/1
  Gain1/1 -> Sum4/1
  Normalize Vector2/1(Normalized) -> 3x3 Cross Product2/1
  myMux Fun2/1(y) -> Normalize Vector2/1(Vector)
  Constant1/1 -> myMux Fun2/3(u3)
  Demux1/2 -> myMux Fun2/2(u2)
  Demux1/1 -> myMux Fun2/1(u1)
  Submatrix1/1 -> Demux1/1
  Sum1/1 -> q dot calc/2(om_hat), Integer Delay/1  "om_hat"
  q dot calc/1(q_dot) -> Discrete-Time Integrator1/1
  Submatrix/1 -> 3x3 Cross Product/2  "g_hat"
  Sum4/1 -> Gain/1, 3D Filter/1(In1)
  3x3 Cross Product1/1 -> Add/1
  A_sens/1 -> Add/3
  Normalize Vector1/1(Normalized) -> 3x3 Cross Product/1
  3x3 Cross Product/1 -> Sum4/2
  Quaternions to  Direction Cosine Matrix/1 -> Submatrix1/1, Product2/1, Product1/1, Submatrix/1, RL2B/1, Direction Cosine Matrix to Rotation Angles/1  "RLT2B"
  Integer Delay/1 -> 3x3 Cross Product1/1
  Discrete-Time Integrator1/1 -> Quaternion Normalize/1  "q1"
  Quaternion Normalize/1 -> Quaternions to  Direction Cosine Matrix/1, q dot calc/1(q)
  "Deriv "/1(ydot) -> Add/2
  Add/1 -> Normalize Vector1/1(Vector)
  acc_bias/1 -> Add/4
  Product1/1 -> 3x3 Cross Product1/2, "Deriv "/1(y)
  Vxyd_hat/1 -> Product1/2
  3D Filter/1(Out1) -> Bias Rate Limiter/1
  Gyros/1 -> Sum3/1
  Gain/1 -> Sum1/2
  Sum3/1 -> Sum1/1, pqr_hat/1  "Gyro Err"
  XY Orient/1 -> 3x3 Cross Product2/2
  3x3 Cross Product2/1 -> Product2/2
  Demux/1 -> Embedded MATLAB Function/1(u)
  Mux/1 -> euler_hat/1
  Embedded MATLAB Function/1(y) -> Mux/3
  Direction Cosine Matrix to Rotation Angles/1 -> Data Type Conversion/1
  Demux/2 -> Mux/2
  Demux/3 -> Mux/1
  Data Type Conversion/1 -> Demux/1
  Demux1/3 -> Terminator10/1

== system AUAV3_WITH_SLUGS_SENSOR_AND_CONTROLLER/Position and Attitude Filter [updated 5.13.16]/COG.SOG2V ==
  COG_D : Inport
  SOG : Inport  Port=2
  Angle Conversion : aerolibconvert2/Angle Conversion  IU=deg  OU=rad
  Constant : Constant  Value=0  OutDataTypeStr=single
  Product : Product  RndMeth=Zero
  Product1 : Product  RndMeth=Zero
  Subsystem5 : Subsystem  AncestorBlock=SLUGS_Library/Subsystem5
  myMux Fun2 : MATLAB Function  TreatAsAtomicUnit=on
  Vnorth : Outport
  Veast : Outport  Port=2
  XY Orient : Outport  Port=3
  wires:
  Product1/1 -> Vnorth/1
  Product/1 -> Veast/1
  SOG/1 -> Product1/1, Product/2
  Angle Conversion/1 -> Subsystem5/1(u)
  Subsystem5/1(sin(u)) -> Product/1, myMux Fun2/2(u2)
  Subsystem5/2(cos(u)) -> Product1/2, myMux Fun2/1(u1)
  COG_D/1 -> Angle Conversion/1
  Constant/1 -> myMux Fun2/3(u3)
  myMux Fun2/1(y) -> XY Orient/1

== system AUAV3_WITH_SLUGS_SENSOR_AND_CONTROLLER/Position and Attitude Filter [updated 5.13.16]/Compute GS Location ==
  GS Location : Inport
  Demux : Demux  Outputs=3
  Geod2ECEF1 : Subsystem  mask{Re=6378137, Rp=6356752.3142}
      mask prompts: Re "Enter equatorial radius, m"; Rp "Enter polar radius,m"
  Mux1 : Mux  Inputs=2
  Mux2 : Mux  Inputs=3
  "Lat, Lon" : Outport
  R_in : Outport  Port=2
  wires:
  Geod2ECEF1/3("Ze, m ") -> Mux2/3
  Geod2ECEF1/1("Xe, m ") -> Mux2/1
  Geod2ECEF1/2("Ye, m ") -> Mux2/2
  Demux/1 -> Geod2ECEF1/1("height, m")
  Demux/2 -> Mux1/2, Geod2ECEF1/2("lat, deg")
  Demux/3 -> Mux1/1, Geod2ECEF1/3(lon,deg)
  GS Location/1 -> Demux/1
  Mux1/1 -> "Lat, Lon"/1
  Mux2/1 -> R_in/1  "R_in"

== system AUAV3_WITH_SLUGS_SENSOR_AND_CONTROLLER/Position and Attitude Filter [updated 5.13.16]/Enabled Subsystem ==
  In1 : Inport
  In2 : Inport  Port=2
  In3 : Inport  Port=3
  Enable : EnablePort
  Out1 : Outport
  Out2 : Outport  Port=2
  Out3 : Outport  Port=3
  wires:
  In1/1 -> Out1/1
  In2/1 -> Out2/1
  In3/1 -> Out3/1

== system AUAV3_WITH_SLUGS_SENSOR_AND_CONTROLLER/Position and Attitude Filter [updated 5.13.16]/GPS Update ==
  XYZ : Inport
  Data Type Conversion2 : DataTypeConversion  OutDataTypeStr=uint8
  Demux : Demux  Outputs=3
  Detect Change : Subsystem
  Detect Change1 : Subsystem
  Detect Change2 : Subsystem
  Rate Transition : RateTransition  OutPortSampleTime=T
  Saturation1 : Saturate  UpperLimit=1  LowerLimit=0  SampleTime=T
  Sum : Sum  Inputs=3
  Update? : Outport
  wires:
  Demux/1 -> Detect Change/1(Data)
  Demux/2 -> Detect Change1/1(Data)
  Demux/3 -> Detect Change2/1(Data)
  Detect Change/1(change?) -> Sum/1
  Detect Change1/1(change?) -> Sum/2
  Detect Change2/1(change?) -> Sum/3
  Sum/1 -> Saturation1/1
  XYZ/1 -> Rate Transition/1
  Saturation1/1 -> Data Type Conversion2/1
  Rate Transition/1 -> Demux/1
  Data Type Conversion2/1 -> Update?/1

== system AUAV3_WITH_SLUGS_SENSOR_AND_CONTROLLER/Position and Attitude Filter [updated 5.13.16]/Geod2LTP1 ==
  GS Lat,Lon : Inport
  GS ECEF : Inport  Port=2
  "Lat, deg(GPS)" : Inport  Port=3
  "Lon, deg(GPS)" : Inport  Port=4
  Hight,m(GPS) : Inport  Port=5
  ECEF2LTP (UEN) : Subsystem
      mask Display: plot(0,0,100,100,[45,40,35,40,40],[85,95,85,95,40],[85,95,85,95,40],[35,40,45,40,40],[60,40,10,20,10,14],[70,40,10,13,10,20],[56,45],[70,70],[60,60],[50,60],[60,60],[30,40],[50,60],[20,20],[30,40],[20,20],[45,55],[35,25],[75,65],[35,25])
  Geod2ECEF1 : Subsystem  mask{Re=6378137, Rp=6356752.3142}
      mask prompts: Re "Enter equatorial radius, m"; Rp "Enter polar radius,m"
  Mux : Mux  Inputs=3
  Reshape : Reshape  OutputDimensionality=Column vector (2-D)
  Reshape1 : Reshape
  Sum1 : Sum  Inputs=|+-  OutDataTypeStr=single  SaturateOnIntegerOverflow=on
  UEN 2 NEU : Gain  Gain=[0 0 1;0 1 0;1 0 0]  Multiplication=Matrix(K*u)  OutDataTypeStr=float('single')  SaturateOnIntegerOverflow=on  ParamDataTypeStr=Inherit: Same as input
  "NEU, m" : Outport
  wires:
  Reshape1/1 -> "NEU, m"/1
  Reshape/1 -> UEN 2 NEU/1
  Sum1/1 -> ECEF2LTP (UEN)/1(ECEF coordinates)
  Mux/1 -> Sum1/1  "r_mov"
  Hight,m(GPS)/1 -> Geod2ECEF1/1("height, m")
  ECEF2LTP (UEN)/1(Out) -> Reshape/1  "Moving Side"
  GS ECEF/1 -> Sum1/2
  GS Lat,Lon/1 -> ECEF2LTP (UEN)/2("Long, Lat")
  "Lon, deg(GPS)"/1 -> Geod2ECEF1/3(lon,deg)
  "Lat, deg(GPS)"/1 -> Geod2ECEF1/2("lat, deg")
  Geod2ECEF1/2("Ye, m ") -> Mux/2
  Geod2ECEF1/1("Xe, m ") -> Mux/1
  Geod2ECEF1/3("Ze, m ") -> Mux/3
  UEN 2 NEU/1 -> Reshape1/1

== system AUAV3_WITH_SLUGS_SENSOR_AND_CONTROLLER/Position and Attitude Filter [updated 5.13.16]/Position Filter [updated 5.13.16] ==
  NewGPS : Inport
  Baro Alt : Inport  Port=2
  RLT2B : Inport  Port=3
  GPS_XYD : Inport  Port=4
  Vnorth : Inport  Port=5
  Veast : Inport  Port=6
  SOG : Inport  Port=7
  A_sens(m/s^2) : Inport  Port=8
  Base Height (m) : Inport  Port=9
  BlendPosVel : Subsystem
  Vxyd_hat : Outport
  Pxyd_hat : Outport  Port=2
  acc_bias : Outport  Port=3
  wires:
  BlendPosVel/3(acc_bias) -> acc_bias/1
  BlendPosVel/1(Vxyd_hat) -> Vxyd_hat/1
  BlendPosVel/2(Pxyd_hat) -> Pxyd_hat/1
  Baro Alt/1 -> BlendPosVel/4(BaroAlt)
  Veast/1 -> BlendPosVel/3(Veast)
  Vnorth/1 -> BlendPosVel/2(Vnorth)
  NewGPS/1 -> BlendPosVel/6(NewGPS)
  RLT2B/1 -> BlendPosVel/5(RLT2B)
  GPS_XYD/1 -> BlendPosVel/1(GPS_NED)
  SOG/1 -> BlendPosVel/7(SOG)
  A_sens(m/s^2)/1 -> BlendPosVel/8(A_sens(m/s^2))
  Base Height (m)/1 -> BlendPosVel/9(Base Height)

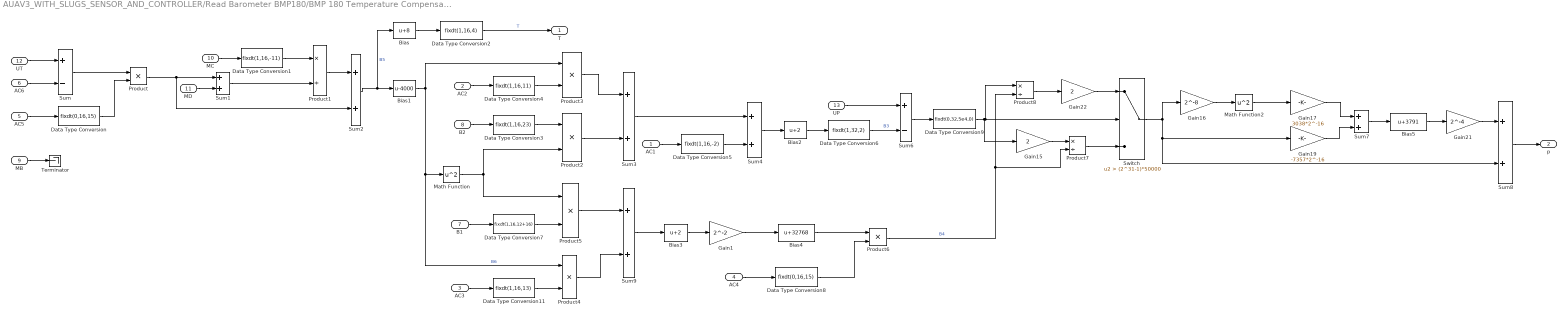
== system AUAV3_WITH_SLUGS_SENSOR_AND_CONTROLLER/Read Barometer BMP180/BMP 180 Temperature Compensation See datasheet ==
  AC1 : Inport
  AC2 : Inport  Port=2
  AC3 : Inport  Port=3
  AC4 : Inport  Port=4
  AC5 : Inport  Port=5
  AC6 : Inport  Port=6
  B1 : Inport  Port=7
  B2 : Inport  Port=8
  MB : Inport  Port=9
  MC : Inport  Port=10
  MD : Inport  Port=11
  UT : Inport  Port=12
  UP : Inport  Port=13
  Bias : Bias  Bias=8
  Bias1 : Bias  Bias=-4000
  Bias2 : Bias  Bias=2
  Bias3 : Bias  Bias=2
  Bias4 : Bias  Bias=32768
  Bias5 : Bias  Bias=3791
  Data Type Conversion : DataTypeConversion  OutDataTypeStr=fixdt(0,16,15)  ConvertRealWorld=Stored Integer (SI)
  Data Type Conversion1 : DataTypeConversion  OutDataTypeStr=fixdt(1,16,-11)  ConvertRealWorld=Stored Integer (SI)
  Data Type Conversion11 : DataTypeConversion  OutDataTypeStr=fixdt(1,16,13)  ConvertRealWorld=Stored Integer (SI)
  Data Type Conversion2 : DataTypeConversion  OutDataTypeStr=fixdt(1,16,4)  ConvertRealWorld=Stored Integer (SI)
  Data Type Conversion3 : DataTypeConversion  OutDataTypeStr=fixdt(1,16,23)  ConvertRealWorld=Stored Integer (SI)
  Data Type Conversion4 : DataTypeConversion  OutDataTypeStr=fixdt(1,16,11)  ConvertRealWorld=Stored Integer (SI)
  Data Type Conversion5 : DataTypeConversion  OutDataTypeStr=fixdt(1,16,-2)  ConvertRealWorld=Stored Integer (SI)
  Data Type Conversion6 : DataTypeConversion  OutDataTypeStr=fixdt(1,32,2)  ConvertRealWorld=Stored Integer (SI)
  Data Type Conversion7 : DataTypeConversion  OutDataTypeStr=fixdt(1,16,12+16)  ConvertRealWorld=Stored Integer (SI)
  Data Type Conversion8 : DataTypeConversion  OutDataTypeStr=fixdt(0,16,15)  ConvertRealWorld=Stored Integer (SI)
  Data Type Conversion9 : DataTypeConversion  OutDataTypeStr=fixdt(0,32,5e4,0)  ConvertRealWorld=Stored Integer (SI)
  Gain1 : Gain  Gain=2^-2  OutDataTypeStr=int32
  Gain15 : Gain  Gain=2  OutDataTypeStr=uint32  RndMeth=Round
  Gain16 : Gain  Gain=2^-8  OutDataTypeStr=int32  RndMeth=Round
  Gain17 : Gain  Gain=3038*2^-16  OutDataTypeStr=uint32
  Gain19 : Gain  Gain=-7357*2^-16  ParamDataTypeStr=fixdt(1,16)  OutDataTypeStr=int32
  Gain21 : Gain  Gain=2^-4  OutDataTypeStr=Inherit: Same as input
  Gain22 : Gain  Gain=2  OutDataTypeStr=Inherit: Same as input
  Math Function : Math  Operator=square  SaturateOnIntegerOverflow=on  OutDataTypeStr=Inherit: Inherit via internal rule
  Math Function2 : Math  Operator=square  OutDataTypeStr=uint32  SaturateOnIntegerOverflow=on
  Product : Product  RndMeth=Round  OutDataTypeStr=Inherit: Same as first input
  Product1 : Product  Inputs=*/  OutDataTypeStr=int16  RndMeth=Round
  Product2 : Product  OutDataTypeStr=int16
  Product3 : Product  OutDataTypeStr=Inherit: Same as first input
  Product4 : Product  OutDataTypeStr=int16
  Product5 : Product  OutDataTypeStr=int16
  Product6 : Product  OutDataTypeStr=uint32
  Product7 : Product  Inputs=*/  RndMeth=Round
  Product8 : Product  Inputs=*/  OutDataTypeStr=uint32  RndMeth=Round
  Sum : Sum  Inputs=+-  RndMeth=Round
  Sum1 : Sum  RndMeth=Round  OutDataTypeStr=Inherit: Same as first input
  Sum2 : Sum  AccumDataTypeStr=int16  OutDataTypeStr=int16  RndMeth=Round
  Sum3 : Sum
  Sum4 : Sum  OutDataTypeStr=int32
  Sum6 : Sum  Inputs=+-  AccumDataTypeStr=uint32  OutDataTypeStr=uint32
  Sum7 : Sum  AccumDataTypeStr=int32  OutDataTypeStr=int32
  Sum8 : Sum  AccumDataTypeStr=int32  OutDataTypeStr=Inherit: Same as accumulator  RndMeth=Round
  Sum9 : Sum
  Switch : Switch  Criteria=u2 > Threshold  Threshold=(2^31-1)*50000
  Terminator : Terminator
  T : Outport
  p : Outport  Port=2
  wires:
  MB/1 -> Terminator/1
  Sum9/1 -> Bias3/1
  Product4/1 -> Sum9/2
  Product5/1 -> Sum9/1
  Product2/1 -> Sum3/2
  Product3/1 -> Sum3/1
  Data Type Conversion3/1 -> Product2/1
  Data Type Conversion11/1 -> Product4/2
  Product1/1 -> Sum2/1
  Data Type Conversion8/1 -> Product6/2
  Data Type Conversion7/1 -> Product5/2
  Data Type Conversion4/1 -> Product3/2
  Math Function/1 -> Product5/1, Product2/2
  Data Type Conversion/1 -> Product/2
  Bias5/1 -> Gain21/1
  Sum8/1 -> p/1
  Gain21/1 -> Sum8/1
  Sum7/1 -> Bias5/1
  Gain17/1 -> Sum7/1
  Gain19/1 -> Sum7/2
  Math Function2/1 -> Gain17/1
  Gain16/1 -> Math Function2/1
  Switch/1 -> Gain19/1, Sum8/2, Gain16/1
  Product7/1 -> Switch/3
  Product8/1 -> Gain22/1
  Data Type Conversion9/1 -> Gain15/1, Product8/1, Switch/2
  Sum6/1 -> Data Type Conversion9/1
  UP/1 -> Sum6/1
  Data Type Conversion6/1 -> Sum6/2  "B3"
  Product6/1 -> Product8/2, Product7/2  "B4"
  Bias4/1 -> Product6/1
  AC4/1 -> Data Type Conversion8/1
  Gain1/1 -> Bias4/1
  Bias3/1 -> Gain1/1
  B1/1 -> Data Type Conversion7/1
  AC3/1 -> Data Type Conversion11/1
  Sum4/1 -> Bias2/1
  Data Type Conversion5/1 -> Sum4/2
  Bias2/1 -> Data Type Conversion6/1
  AC1/1 -> Data Type Conversion5/1
  Sum3/1 -> Sum4/1
  AC2/1 -> Data Type Conversion4/1
  B2/1 -> Data Type Conversion3/1
  Bias1/1 -> Product3/1, Product4/1, Math Function/1  "B6"
  MC/1 -> Data Type Conversion1/1
  Data Type Conversion2/1 -> T/1  "T"
  Bias/1 -> Data Type Conversion2/1
  Sum1/1 -> Product1/2
  Sum2/1 -> Bias1/1, Bias/1  "B5"
  Product/1 -> Sum1/1, Sum2/2
  MD/1 -> Sum1/2
  AC5/1 -> Data Type Conversion/1
  Sum/1 -> Product/1
  AC6/1 -> Sum/2
  UT/1 -> Sum/1
  Data Type Conversion1/1 -> Product1/1
  Gain22/1 -> Switch/1
  Gain15/1 -> Product7/1
